simulink model "W02_C_metrics"  (R2024b)
settings: Solver=ode4  StartTime=0  StopTime=T_final  FixedStep=h  RelTol=1e-3
values from neighbouring files (symbols this model uses):
  Kp = 10    [W02_0_setup.m]    (also in W02_D_derivative.m; W02_E_integral.m; W02_I_tuning_by_hand.m = 5*k)
  pid_b = 2    [W02_0_setup.m]
  pid_k = 2    [W02_0_setup.m]
  pid_m = 1    [W02_0_setup.m]
  t_step = 1    [W02_0_setup.m]
  y_step = 1    [W02_0_setup.m]
settings Model: Creator=admin  LastModifiedBy=admin
settings DataIOCC: ReturnWorkspaceOutputs=off

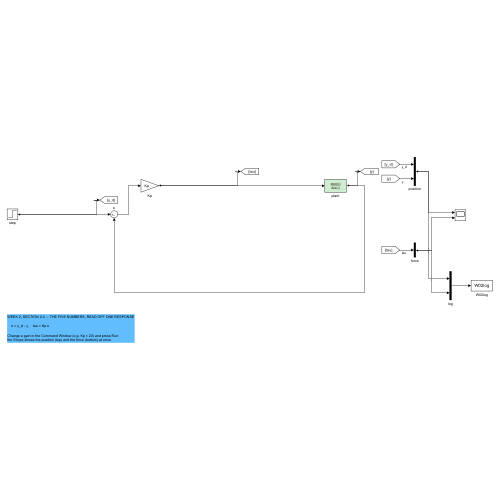
[thumbnail: Simulink's stored preview of the top-level diagram]
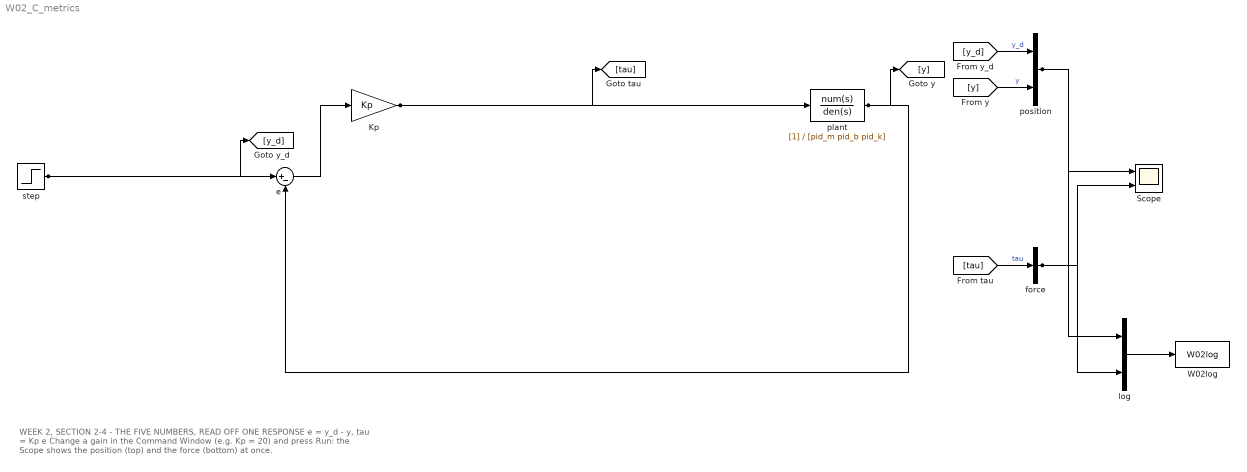
== system W02_C_metrics ==
  note: WEEK 2, SECTION 2-4  -  THE FIVE NUMBERS, READ OFF ONE RESPONSE
      |
      |     e = y_d - y,    tau = Kp e
      |
      | Change a gain in the Command Window (e.g. Kp = 20) and press Run:
      | the Scope shows the position (top) and the force (bottom) at once.
  Kp : Gain  Gain=Kp
  Scope : Scope  NumInputPorts=2
  W02log : ToWorkspace  VariableName=W02log  SaveFormat=Structure With Time  SampleTime=-1
  e : Sum  Inputs=|+-
  force : Mux  Inputs=1
  log : Mux  Inputs=2
  plant : TransferFcn  Denominator=[pid_m pid_b pid_k]
  position : Mux  Inputs=2
  step : Step  Time=t_step  After=y_step  SampleTime=0
  wires:
  step/1 -> e/1, [y_d]
  e/1 -> Kp/1
  Kp/1 -> plant/1, [tau]
  plant/1 -> [y], e/2
  [y_d] -> position/1  "y_d"
  [y] -> position/2  "y"
  [tau] -> force/1  "tau"
  position/1 -> Scope/1, log/1
  force/1 -> Scope/2, log/2
  log/1 -> W02log/1
